simulink subsystem "FIFO_Serializer"  (R2024a)
settings: Solver=VariableStepAuto  StartTime=0.0  StopTime=10.0  RelTol=1e-3
model mask{FIFOLength=0}
libraries: hdlsllib x3, simulink x1
settings Model: Creator=versal  LastModifiedBy=versal

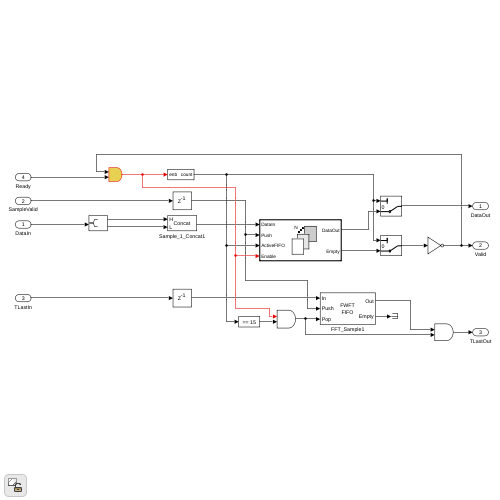
[thumbnail: Simulink's stored preview of the top-level diagram]
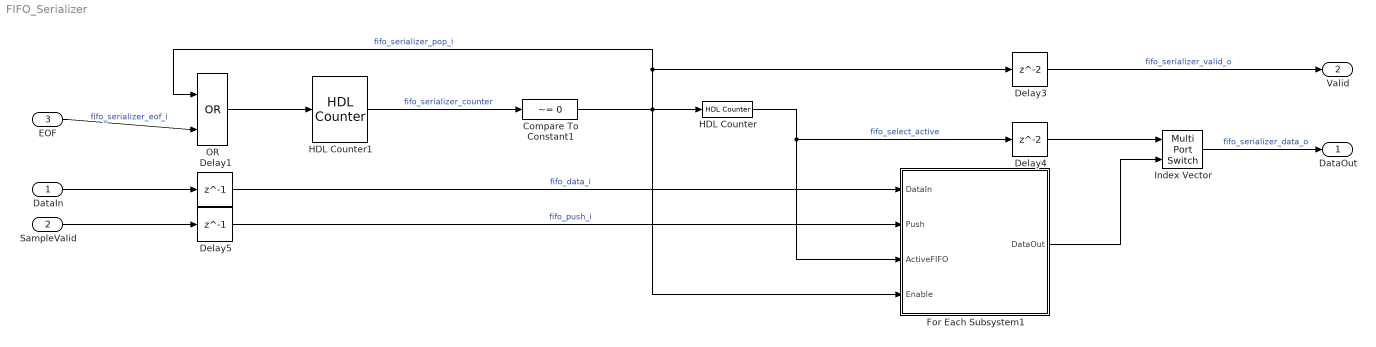
== system FIFO_Serializer ==
  DataIn : Inport
  SampleValid : Inport  Port=2
  EOF : Inport  Port=3
  Compare To Constant1 : simulink/Logic and Bit Operations/Compare To Constant  relop=~=  const=0  OutDataTypeStr=boolean
  Delay1 : Delay  DelayLength=1
  Delay3 : Delay
  Delay4 : Delay
  Delay5 : Delay  DelayLength=1
  For Each Subsystem1 : Subsystem  TreatAsAtomicUnit=on
  HDL Counter : hdlsllib/Sources/HDL Counter  CountType=Count limited  CountInit=0  CountStep=1  CountMax=3  CountFromType=Initial value  CountFrom=0  CountResetPort=off  CountLoadPort=off  CountEnbPort=on  CountDirPort=off  CountHitOutputPort=off  CountDataType=Unsigned  CountWordLen=3  CountFracLen=0  CountSampTime=1
  HDL Counter1 : hdlsllib/Sources/HDL Counter  CountType=Count limited  CountInit=0  CountStep=1  CountMax=256  CountFromType=Initial value  CountFrom=0  CountResetPort=off  CountLoadPort=off  CountEnbPort=on  CountDirPort=off  CountHitOutputPort=off  CountDataType=Unsigned  CountWordLen=9  CountFracLen=0  CountSampTime=1
  Index Vector : MultiPortSwitch  DataPortOrder=Zero-based contiguous  Inputs=1  zeroidx=on  SaturateOnIntegerOverflow=off  InputSameDT=off
  OR : Logic  Operator=OR  IconShape=distinctive  AllPortsSameDT=off  OutDataTypeStr=boolean
  DataOut : Outport  VectorParamsAs1DForOutWhenUnconnected=off
  Valid : Outport  Port=2  VectorParamsAs1DForOutWhenUnconnected=off
  wires:
  SampleValid/1 -> Delay5/1
  For Each Subsystem1/1(DataOut) -> Index Vector/2
  EOF/1 -> OR/2  "fifo_serializer_eof_i"
  Delay5/1 -> For Each Subsystem1/2(Push)  "fifo_push_i"
  DataIn/1 -> Delay1/1
  Delay1/1 -> For Each Subsystem1/1(DataIn)  "fifo_data_i"
  OR/1 -> HDL Counter1/1
  HDL Counter1/1 -> Compare To Constant1/1  "fifo_serializer_counter"
  Compare To Constant1/1 -> HDL Counter/1, Delay3/1, OR/1, For Each Subsystem1/4(Enable)  "fifo_serializer_pop_i"
  Index Vector/1 -> DataOut/1  "fifo_serializer_data_o"
  Delay3/1 -> Valid/1  "fifo_serializer_valid_o"
  HDL Counter/1 -> For Each Subsystem1/3(ActiveFIFO), Delay4/1  "fifo_select_active"
  Delay4/1 -> Index Vector/1

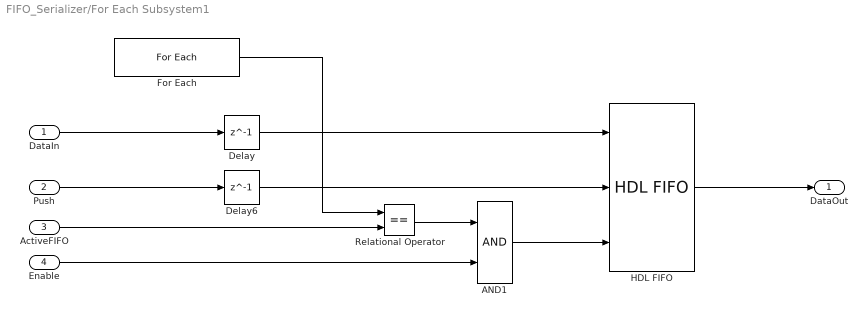
== system FIFO_Serializer/For Each Subsystem1 ==
  DataIn : Inport  Partition=on  PartitionDimension=2  PartitionWidth=1  PartitionOffset=0
  Push : Inport  Port=2
  ActiveFIFO : Inport  Port=3
  Enable : Inport  Port=4
  AND1 : Logic  IconShape=distinctive  AllPortsSameDT=off  OutDataTypeStr=boolean
  Delay : Delay  DelayLength=1
  Delay6 : Delay  DelayLength=1
  For Each : ForEach  DisableCoverage=on  ShowIterationIndex=on
  HDL FIFO : hdlsllib/HDL RAMs/HDL FIFO  fifo_size=70  mode=FWFT  ratio=1  push_msg=Warning  pop_msg=Warning  show_empty=off  show_full=off  show_num=off  LabelModeActiveChoice_Mode=FWFT  rst_port=off
  Relational Operator : RelationalOperator  Operator===  OutDataTypeStr=boolean  RndMeth=Simplest  InputSameDT=off
  DataOut : Outport  ConcatenationDimension=1
  wires:
  DataIn/1 -> Delay/1
  AND1/1 -> HDL FIFO/3
  Delay/1 -> HDL FIFO/1
  Delay6/1 -> HDL FIFO/2
  For Each/1 -> Relational Operator/1
  HDL FIFO/1 -> DataOut/1
  Push/1 -> Delay6/1
  Relational Operator/1 -> AND1/1
  ActiveFIFO/1 -> Relational Operator/2
  Enable/1 -> AND1/2
